simulink model "pendulum_model"  (R2025b)
settings: Solver=FixedStepAuto  StartTime=0.0  StopTime=20  FixedStep=0.01  RelTol=1e-3
values from neighbouring files (symbols this model uses):
  G_fii = -0.008456    [run_simulink_model.m]
  G_t = 4.097306    [run_simulink_model.m]
  G_tp = -0.152144    [run_simulink_model.m]
  Gfi = -1.045953    [run_simulink_model.m]
  Gu = 457.443480    (= 457.44348)    [run_simulink_model.m]
  useSignForFrict = 1    [run_simulink_model.m]
  withMotor = 1    [run_simulink_model.m]
  x0_state = [pendVel(1), pendPosZU(1)]    [run_simulink_model.m]
libraries: simulink x1
settings Model: Creator=igorsiata  LastModifiedBy=igorsiata

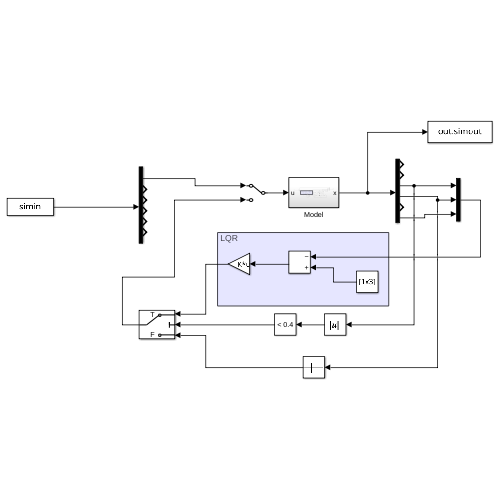
[thumbnail: Simulink's stored preview of the top-level diagram]
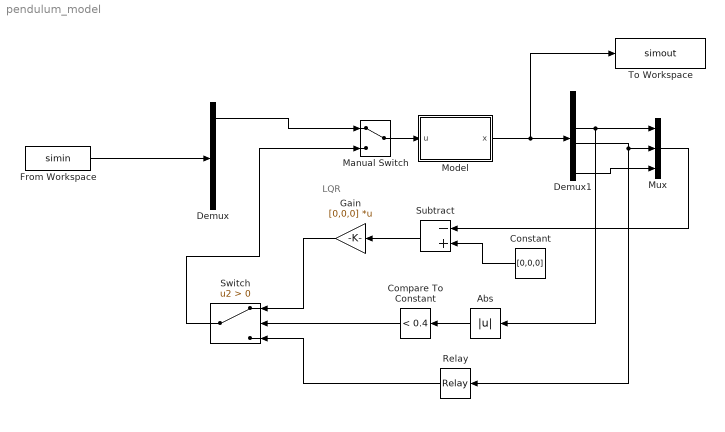
== system pendulum_model ==
  note: LQR
  Abs : Abs  SaturateOnIntegerOverflow=off
  Compare To Constant : simulink/Logic and Bit Operations/Compare To Constant  relop=<  const=0.4  OutDataTypeStr=boolean
  Constant : Constant  Value=[0,0,0]
  Demux : Demux  Outputs=6
  Demux1 : Demux  Outputs=6
  From Workspace : FromWorkspace  VariableName=simin
  Gain : Gain  Gain=[0,0,0]  Multiplication=Matrix(K*u)
  Manual Switch : ManualSwitch
  Model : Subsystem
  Mux : Mux  Inputs=3
  Relay : Relay  OnSwitchValue=0  OffSwitchValue=0  OnOutputValue=-0.5  OffOutputValue=0.5
  Subtract : Sum  Inputs=-+
  Switch : Switch  Criteria=u2 > Threshold  SaturateOnIntegerOverflow=off  InputSameDT=off
  To Workspace : ToWorkspace  VariableName=simout  SaveFormat=Timeseries  SampleTime=-1
  wires:
  From Workspace/1 -> Demux/1
  Model/1(x) -> To Workspace/1, Demux1/1
  Demux1/3 -> Abs/1, Mux/1
  Demux1/4 -> Relay/1, Mux/2
  Demux1/6 -> Mux/3
  Manual Switch/1 -> Model/1(u)
  Abs/1 -> Compare To Constant/1
  Compare To Constant/1 -> Switch/2
  Switch/1 -> Manual Switch/2
  Demux/1 -> Manual Switch/1
  Relay/1 -> Switch/3
  Gain/1 -> Switch/1
  Mux/1 -> Subtract/1
  Subtract/1 -> Gain/1
  Constant/1 -> Subtract/2

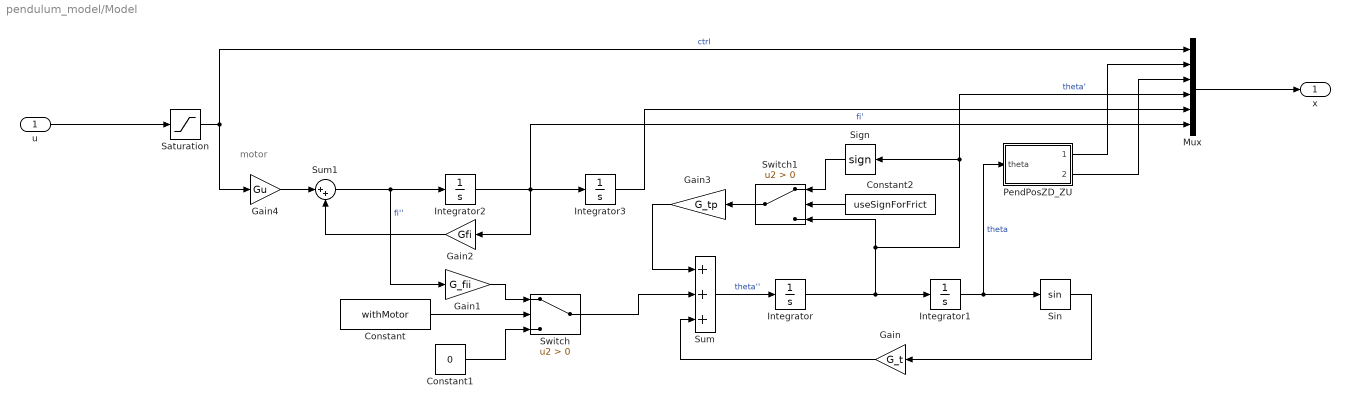
== system pendulum_model/Model ==
  note: motor
  u : Inport
  Constant : Constant  Value=withMotor
  Constant1 : Constant  Value=0
  Constant2 : Constant  Value=useSignForFrict
  Gain : Gain  Gain=G_t
  Gain1 : Gain  Gain=G_fii
  Gain2 : Gain  Gain=Gfi
  Gain3 : Gain  Gain=G_tp
  Gain4 : Gain  Gain=Gu
  Integrator : Integrator  InitialCondition=x0_state(1)
  Integrator1 : Integrator  InitialCondition=x0_state(2)
  Integrator2 : Integrator
  Integrator3 : Integrator
  Mux : Mux  Inputs=6
  PendPosZD_ZU : Subsystem
  Saturation : Saturate  UpperLimit=1  LowerLimit=-1
  Sign : Signum
  Sin : Trigonometry
  Sum : Sum  Inputs=+++
  Sum1 : Sum  Inputs=|++
  Switch : Switch  Criteria=u2 > Threshold  SaturateOnIntegerOverflow=off  InputSameDT=off
  Switch1 : Switch  Criteria=u2 > Threshold  SaturateOnIntegerOverflow=off  InputSameDT=off
  x : Outport
  wires:
  Sum/1 -> Integrator/1  "theta''"
  Constant/1 -> Switch/2
  Constant2/1 -> Switch1/2
  Mux/1 -> x/1
  Gain3/1 -> Sum/1
  Integrator1/1 -> PendPosZD_ZU/1(theta), Sin/1  "theta"
  Sign/1 -> Switch1/1
  Integrator/1 -> Mux/4, Sign/1, Switch1/3, Integrator1/1  "theta'"
  u/1 -> Saturation/1
  Sin/1 -> Gain/1
  Gain1/1 -> Switch/1
  Constant1/1 -> Switch/3
  Switch1/1 -> Gain3/1
  Integrator3/1 -> Mux/5
  Sum1/1 -> Gain1/1, Integrator2/1  "fi''"
  Integrator2/1 -> Integrator3/1, Mux/6, Gain2/1  "fi'"
  Saturation/1 -> Mux/1, Gain4/1  "ctrl"
  Gain4/1 -> Sum1/1
  Gain2/1 -> Sum1/2
  Gain/1 -> Sum/3
  Switch/1 -> Sum/2
  PendPosZD_ZU/1(PendPosZD) -> Mux/2
  PendPosZD_ZU/2(PendPosZU) -> Mux/3

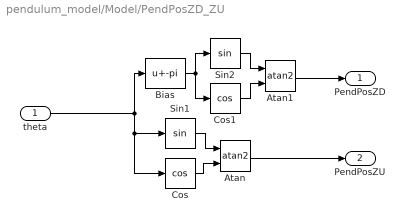
== system pendulum_model/Model/PendPosZD_ZU ==
  theta : Inport
  Atan : Trigonometry  Operator=atan2
  Atan1 : Trigonometry  Operator=atan2
  Bias : Bias  Bias=-pi  SaturateOnIntegerOverflow=off
  Cos : Trigonometry  Operator=cos
  Cos1 : Trigonometry  Operator=cos
  Sin1 : Trigonometry
  Sin2 : Trigonometry
  PendPosZD : Outport
  PendPosZU : Outport  Port=2
  wires:
  Sin2/1 -> Atan1/1
  Atan/1 -> PendPosZU/1
  Cos/1 -> Atan/2
  Cos1/1 -> Atan1/2
  Bias/1 -> Cos1/1, Sin2/1
  Sin1/1 -> Atan/1
  theta/1 -> Cos/1, Sin1/1, Bias/1
  Atan1/1 -> PendPosZD/1
